simulink model "main"  (R2020b)
settings: Solver=VariableStepAuto  StartTime=0.0  StopTime=Inf  RelTol=1e-3
settings Model: Creator=Usuario  LastModifiedBy=Usuario

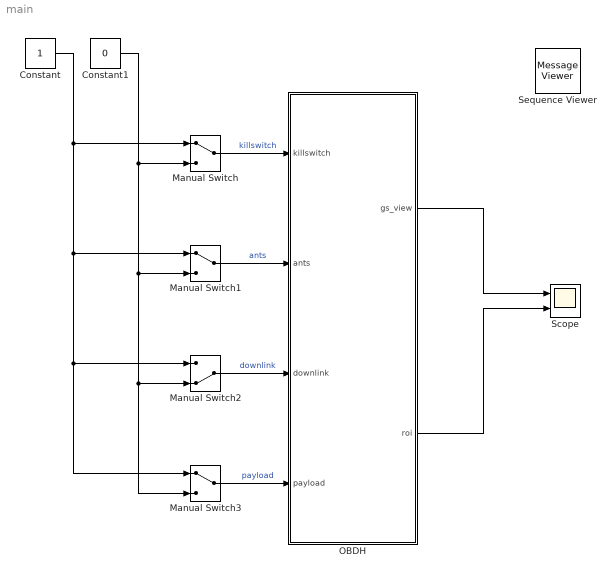
== system main ==
  Constant : Constant
  Constant1 : Constant  Value=0
  Manual Switch : ManualSwitch
  Manual Switch1 : ManualSwitch
  Manual Switch2 : ManualSwitch  CurrentSetting=0
  Manual Switch3 : ManualSwitch
  OBDH : Stateflow chart  TreatAsAtomicUnit=on
  Scope : Scope  NumInputPorts=2
  Sequence Viewer : MessageViewer
  wires:
  Constant/1 -> Manual Switch3/1, Manual Switch2/1, Manual Switch1/1, Manual Switch/1
  Constant1/1 -> Manual Switch3/2, Manual Switch2/2, Manual Switch1/2, Manual Switch/2
  Manual Switch/1 -> OBDH/1(killswitch)  "killswitch"
  Manual Switch1/1 -> OBDH/2(ants)  "ants"
  Manual Switch2/1 -> OBDH/3(downlink)  "downlink"
  Manual Switch3/1 -> OBDH/4(payload)  "payload"
  OBDH/1(gs_view) -> Scope/1
  OBDH/2(roi) -> Scope/2

== stateflow chart main/OBDH ==
  state off
  state boot
  state operational
    state idle
    state downlink
    state payload
    (default) -> idle
    idle -> downlink [order 1] : [downlink==1]{gs_view=1}
    idle -> payload [order 2] : [payload==1]{roi=1}
    downlink -> idle : [downlink ==0]{gs_view=0}
    payload -> idle : [payload==0]{roi=0}
  (default) -> off
  off -> boot : [killswitch==1]
  boot -> operational : [ants==1]
  data: killswitch input; ants input; downlink input; payload input; gs_view output; roi output
